simulink model "Model_witch_OPC_comm"  (R2022b)
settings: Solver=FixedStepDiscrete  StartTime=0.0  StopTime=inf  FixedStep=Ts  RelTol=1e-3  EnableMultiTasking=on
model workspace (MAT data in the model file):
  Param = Simulink.Parameter
  Param.DataType = 'auto'
  Param.Complexity = 'real'
  Param.Dimensions = [0 0]
  Param1 = Simulink.Parameter
  Param1.DataType = 'auto'
  Param1.Complexity = 'real'
  Param1.Dimensions = [0 0]
  Ts = Simulink.Parameter
  Ts.Value = 0.02
  Ts.DataType = 'double'
  Ts.Complexity = 'real'
  Ts.Dimensions = [1 1]
  Var = 0
  c = Simulink.Parameter
  c.Value = 1
  c.DataType = 'double'
  c.Complexity = 'real'
  c.Dimensions = [1 1]
  g = Simulink.Parameter
  g.Value = 9.81
  g.DataType = 'double'
  g.Complexity = 'real'
  g.Dimensions = [1 1]
  l = Simulink.Parameter
  l.Value = 0.75
  l.DataType = 'double'
  l.Complexity = 'real'
  l.Dimensions = [1 1]
  m = Simulink.Parameter
  m.Value = 2
  m.DataType = 'double'
  m.Complexity = 'real'
  m.Dimensions = [1 1]
  pi = Simulink.Parameter
  pi.Value = 3.14
  pi.DataType = 'double'
  pi.Complexity = 'real'
  pi.Dimensions = [1 1]
undefined symbols (not defined in the file or in its folder): DiscIntNeverNeededParam
libraries: opclib x1
settings Model: Creator=siemens  LastModifiedBy=kerif
settings SolverCC: AlgebraicLoopSolver=TrustRegion
settings DataIOCC: LimitDataPoints=on  SaveFormat=Array  ReturnWorkspaceOutputs=off
settings OptimizationCC: LifeSpan=inf
settings DebuggingCC: SolverPrmCheckMsg=warning  UnconnectedInputMsg=warning  UnconnectedOutputMsg=warning  UnconnectedLineMsg=warning  SFUnexpectedBacktrackingDiag=warning  SFNoUnconditionalDefaultTransitionDiag=warning  SFMachineParentedDataDiag=warning  ArithmeticOperatorsInVariantConditions=warning
settings HardwareCC: ProdBitPerPointer=32  ProdBitPerSizeT=32  ProdBitPerPtrDiffT=32  ProdLargestAtomicFloat=None  ProdIntDivRoundTo=Undefined  ProdEndianess=Unspecified  ProdWordSize=32  ProdHWDeviceType=32-bit Generic
settings ModelReferenceCC: EnableRefExpFcnMdlSchedulingChecks=on  PropagateSignalLabelsOutOfModel=off
settings SFSimCC: SimUseLocalCustomCode=off  CustomCodeUndefinedFunction=UseInterfaceOnly
settings RTWCC: RTWUseLocalCustomCode=off  DLArmComputeVersion=19.05
settings CodeAppCC: StateflowObjectComments=on
settings GRTTargetCC: TargetLangStandard=C89/C90 (ANSI)
settings ConfigComp: CovMetricSettings=dw  CovSaveCumulativeToWorkspaceVar=on  CovSaveSingleToWorkspaceVar=on  CovExternalEMLEnable=off  CovSFcnEnable=off

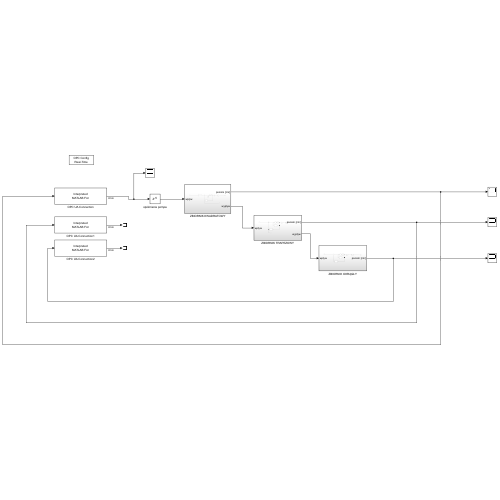
[thumbnail: Simulink's stored preview of the top-level diagram]
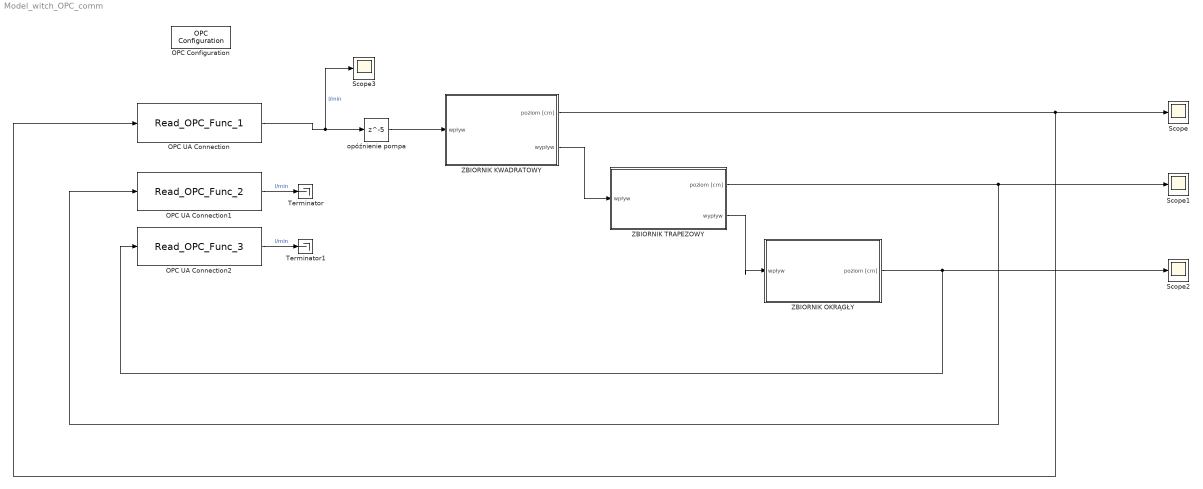
== system Model_witch_OPC_comm ==
  OPC Configuration : opclib/OPC Configuration  opcServers=localhost/opc.tcp://192.168.1.100:4840/10  errMissingItems=Error  errReadWrite=Warn  errShutdown=Error  errRTViolation=Warn  rtEnable=on  speedup=1  showLatency=off  beingUsed=on
  OPC UA Connection : MATLABFcn  MATLABFcn=Read_OPC_Func_1  OutputDimensions=1  OutputSignalType=real  Output1D=off
  OPC UA Connection1 : MATLABFcn  MATLABFcn=Read_OPC_Func_2  OutputDimensions=1  OutputSignalType=real  Output1D=off
  OPC UA Connection2 : MATLABFcn  MATLABFcn=Read_OPC_Func_3  OutputDimensions=1  OutputSignalType=real  Output1D=off
  Scope{,1..3} (4 alike) : Scope
  Terminator : Terminator
  Terminator1 : Terminator
  ZBIORNIK KWADRATOWY : Subsystem
  ZBIORNIK OKRĄGŁY : Subsystem
  ZBIORNIK TRAPEZOWY : Subsystem
  opóźnienie pompa : Delay  DelayLength=5
  wires:
  ZBIORNIK KWADRATOWY/1(poziom [cm]) -> OPC UA Connection/1, Scope/1
  ZBIORNIK TRAPEZOWY/1(poziom [cm]) -> Scope1/1, OPC UA Connection1/1
  ZBIORNIK KWADRATOWY/2(wypływ) -> ZBIORNIK TRAPEZOWY/1(wpływ)
  ZBIORNIK TRAPEZOWY/2(wypływ) -> ZBIORNIK OKRĄGŁY/1(wpływ)
  ZBIORNIK OKRĄGŁY/1(poziom [cm]) -> OPC UA Connection2/1, Scope2/1
  opóźnienie pompa/1 -> ZBIORNIK KWADRATOWY/1(wpływ)
  OPC UA Connection/1 -> Scope3/1, opóźnienie pompa/1  "l/min"
  OPC UA Connection1/1 -> Terminator/1  "l/min"
  OPC UA Connection2/1 -> Terminator1/1  "l/min"

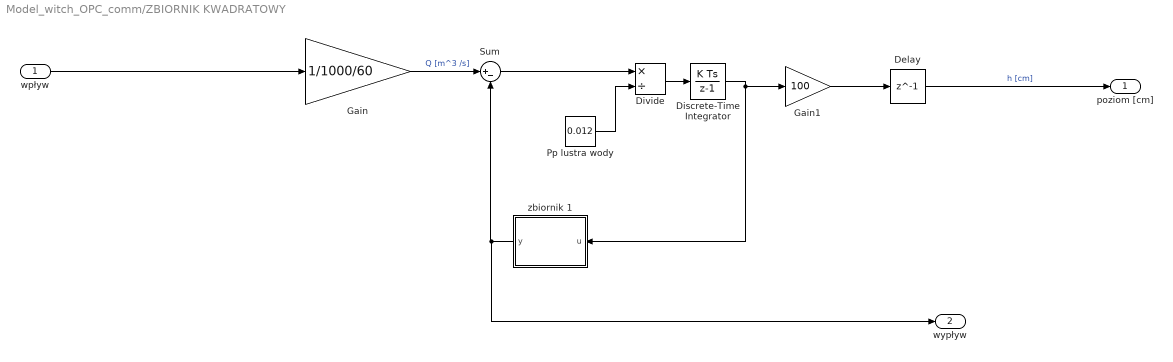
== system Model_witch_OPC_comm/ZBIORNIK KWADRATOWY ==
  wpływ : Inport
  Delay : Delay  DelayLength=1  InitialCondition=0
  Discrete-Time Integrator : DiscreteIntegrator  InitialCondition=0.00000001  SampleTime=Ts  LimitOutput=on  UpperSaturationLimit=0.3  LowerSaturationLimit=0.0000000001  ICPrevOutput=DiscIntNeverNeededParam  ICPrevScaledInput=DiscIntNeverNeededParam
  Divide : Product  Inputs=*/
  Gain : Gain  Gain=1/1000/60
  Gain1 : Gain  Gain=100
  Pp lustra wody : Constant  Value=0.012
  Sum : Sum  Inputs=|+-
  zbiornik 1 : MATLAB Function  TreatAsAtomicUnit=on
  poziom [cm] : Outport
  wypływ : Outport  Port=2
  wires:
  Divide/1 -> Discrete-Time Integrator/1
  zbiornik 1/1(y) -> wypływ/1, Sum/2
  Gain1/1 -> Delay/1
  Discrete-Time Integrator/1 -> zbiornik 1/1(u), Gain1/1
  Gain/1 -> Sum/1  "Q [m^3 /s]"
  Sum/1 -> Divide/1
  Pp lustra wody/1 -> Divide/2
  wpływ/1 -> Gain/1
  Delay/1 -> poziom [cm]/1  "h [cm]"

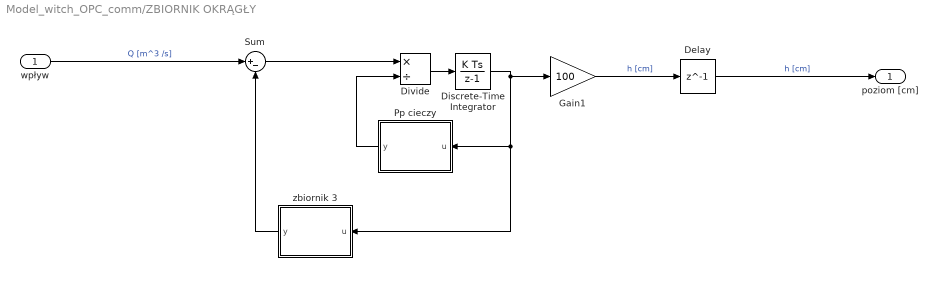
== system Model_witch_OPC_comm/ZBIORNIK OKRĄGŁY ==
  wpływ : Inport
  Delay : Delay  DelayLength=1  InitialCondition=0
  Discrete-Time Integrator : DiscreteIntegrator  InitialCondition=0.0000000001  SampleTime=Ts  LimitOutput=on  UpperSaturationLimit=0.3  LowerSaturationLimit=0.0000000001  ICPrevOutput=DiscIntNeverNeededParam  ICPrevScaledInput=DiscIntNeverNeededParam
  Divide : Product  Inputs=*/
  Gain1 : Gain  Gain=100
  Pp cieczy : MATLAB Function  TreatAsAtomicUnit=on
  Sum : Sum  Inputs=|+-
  zbiornik 3 : MATLAB Function  TreatAsAtomicUnit=on
  poziom [cm] : Outport
  wires:
  Divide/1 -> Discrete-Time Integrator/1
  zbiornik 3/1(y) -> Sum/2
  Discrete-Time Integrator/1 -> Pp cieczy/1(u), zbiornik 3/1(u), Gain1/1
  wpływ/1 -> Sum/1  "Q [m^3 /s]"
  Sum/1 -> Divide/1
  Gain1/1 -> Delay/1  "h [cm]"
  Pp cieczy/1(y) -> Divide/2
  Delay/1 -> poziom [cm]/1  "h [cm]"

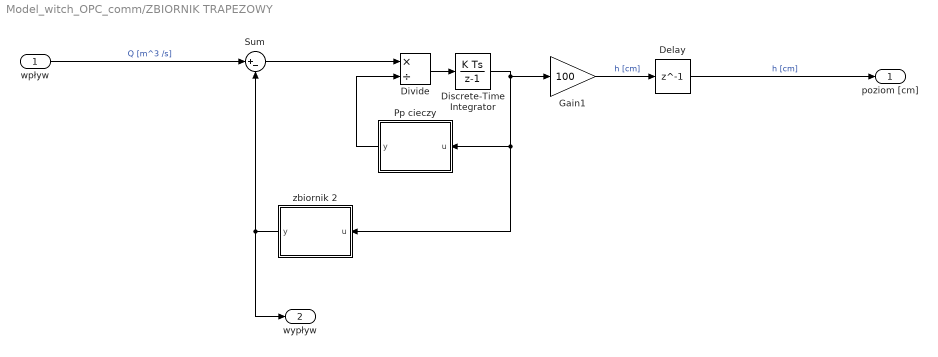
== system Model_witch_OPC_comm/ZBIORNIK TRAPEZOWY ==
  wpływ : Inport
  Delay : Delay  DelayLength=1  InitialCondition=0
  Discrete-Time Integrator : DiscreteIntegrator  InitialCondition=0.0000000001  SampleTime=Ts  LimitOutput=on  UpperSaturationLimit=0.3  LowerSaturationLimit=0.0000000001  ICPrevOutput=DiscIntNeverNeededParam  ICPrevScaledInput=DiscIntNeverNeededParam
  Divide : Product  Inputs=*/
  Gain1 : Gain  Gain=100
  Pp cieczy : MATLAB Function  TreatAsAtomicUnit=on
  Sum : Sum  Inputs=|+-
  zbiornik 2 : MATLAB Function  TreatAsAtomicUnit=on
  poziom [cm] : Outport
  wypływ : Outport  Port=2
  wires:
  Divide/1 -> Discrete-Time Integrator/1
  zbiornik 2/1(y) -> Sum/2, wypływ/1
  Discrete-Time Integrator/1 -> Pp cieczy/1(u), zbiornik 2/1(u), Gain1/1
  wpływ/1 -> Sum/1  "Q [m^3 /s]"
  Sum/1 -> Divide/1
  Gain1/1 -> Delay/1  "h [cm]"
  Pp cieczy/1(y) -> Divide/2
  Delay/1 -> poziom [cm]/1  "h [cm]"

== matlab function Model_witch_OPC_comm/ZBIORNIK KWADRATOWY/zbiornik 1 ==
  data: u input; y output
function y = fcn(u)


 y = 0.63*sqrt(2*9.81*u)*pi*(1/100)^2;

== matlab function Model_witch_OPC_comm/ZBIORNIK TRAPEZOWY/Pp cieczy ==
  data: u input; y output
function y = fcn(u)


 y = (0.2/0.3)*u + 0.008;

== matlab function Model_witch_OPC_comm/ZBIORNIK OKRĄGŁY/Pp cieczy ==
  data: u input; y output
function y = fcn(u)


 y = (sqrt(0.2^2-(0.2-u)^2)+0.2)*0.04;

== matlab function Model_witch_OPC_comm/ZBIORNIK OKRĄGŁY/zbiornik 3 ==
  data: u input; y output
function y = fcn(u)

y = 0.63*sqrt(2*9.81*u)*pi*(1/100)^2;

== matlab function Model_witch_OPC_comm/ZBIORNIK TRAPEZOWY/zbiornik 2 ==
  data: u input; y output
function y = fcn(u)

y = 0.63*sqrt(2*9.81*u)*pi*(1/100)^2;
